simulink library "modbus_lib"  (R2016b)
settings: Solver=ode45  StartTime=0.0  StopTime=10.0  RelTol=1e-3  EnableMultiTasking=on
undefined symbols (not defined in the file): angle_threshold, dF_threshold, DiscIntNeverNeededParam, dV_threshold, IOC, relay_sets, TOC, Ts, V, VRMSLL
libraries: simulink x21, powerlib_extras x20, powerlib x20, modbus_lib x8, simulink_extras x5, lib_Timer_Counter x4, rtio_generic_modbus x3, simulink_need_slupdate x3, dspsigops x2, discreteBreakerBlock x1
(part 1 of 2)
settings Model: Creator=RE25624  LastModifiedBy=ch24070
settings DataIOCC: LimitDataPoints=on  SaveFormat=Array  SignalLoggingSaveFormat=ModelDataLogs
settings OptimizationCC: ExpressionDepthLimit=2147483647  LifeSpan=inf
settings DebuggingCC: UnderspecifiedInitializationDetection=Classic  MergeDetectMultiDrivingBlocksExec=none  SolverPrmCheckMsg=warning  FcnCallInpInsideContextMsg=warning  StateNameClashWarn=warning  SFUnexpectedBacktrackingDiag=warning  SFNoUnconditionalDefaultTransitionDiag=warning  SFExecutionAtInitializationDiag=none
settings HardwareCC: ProdBitPerPointer=32  ProdBitPerSizeT=32  ProdBitPerPtrDiffT=32  ProdLargestAtomicFloat=None  ProdIntDivRoundTo=Undefined  ProdEndianess=Unspecified  ProdWordSize=32  ProdHWDeviceType=32-bit Generic
settings ModelReferenceCC: PropagateSignalLabelsOutOfModel=off
settings GRTTargetCC: TargetLangStandard=C89/C90 (ANSI)  GeneratePreprocessorConditionals=Disable all  CombineOutputUpdateFcns=off  GRTInterface=on
settings ConfigComp: CovMetricSettings=dw  CovHtmlReporting=on  CovSaveCumulativeToWorkspaceVar=on  CovSaveSingleToWorkspaceVar=on  CovExternalEMLEnable=off

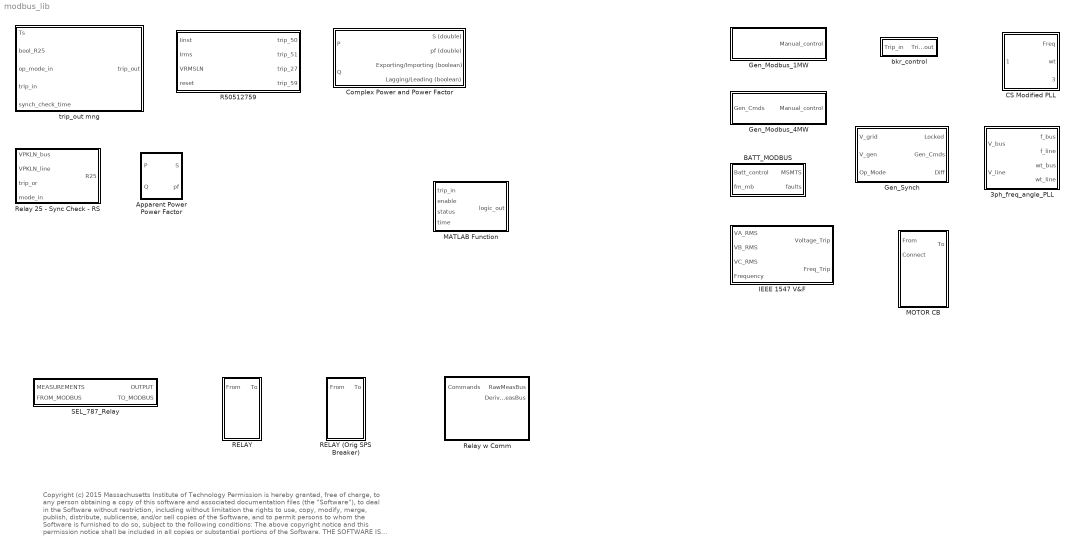
== system modbus_lib ==
  note: Copyright (c) 2015 Massachusetts Institute of Technology
      | Permission is hereby granted, free of charge, to any person obtaining a copy of this software and associated documentation files (the "Software"), to deal in the Software without restriction, including without limitation the rights to use, copy, modify, merge, publish, distribute, sublicense, and/or sell copies of the Software, and to permit persons to whom the Software is furnished to do so, subject to the following conditions:
      |
      | The above copyright notice and this permission notice shall be included in all copies or substantial portions of the Software.
      |
      | THE SOFTWARE IS PROVIDED "AS IS", WITHOUT WARRANTY OF ANY KIND, EXPRESS OR IMPLIED, INCLUDING BUT NOT LIMITED TO THE WARRANTIES OF MERCHANTABILITY, FITNESS FOR A PARTICULAR PURPOSE AND NONINFRINGEMENT. IN NO EVENT SHALL THE AUTHORS OR COPYRIGHT HOLDERS BE LIABLE FOR ANY CLAIM,
      | DAMAGES OR OTHER LIABILITY, WHETHER IN AN ACTION OF CONTRACT, TORT OR OTHERWISE, ARISING FROM, OUT OF OR IN CONNECTION WITH THE SOFTWARE OR THE USE OR OTHER DEALINGS IN THE SOFTWARE.
  3ph_freq_angle_PLL : Subsystem
  Apparent Power Power Factor : Subsystem
  BATT_MODBUS : Subsystem
  CS Modified PLL : Subsystem  DialogController=POWERSYS.PowerSysDialog  mask(Discrete 3-phase PLL){Fmin=50, Par_Init=[0 60], ParK=[ 180 3200 1 ], Ts=Ts, AGC=off}
      mask prompts: Fmin "Minimum frequency (Hz):"; Par_Init "Initial inputs:[ Phase(degrees)   Frequency(Hz) ]"; ParK "Regulator gains [ Kp  Ki  Kd ]"; Ts "Sample time:"; AGC "Enable Automatic Gain Control"
      mask help:
      | This Phase Locked Loop (PLL) system can be used  to synchronize on a set of variable frequency, three-phase sinusoidal signals. If the Automatic Gain Control is enabled, the input (phase error) of the PLL regulator is scaled according to the input signals magnitude.
      |
      | For optimal performance, the following settings are recommended:
      |   [ Kp Ki  Kd ] = [ 180  3200  1 ]
      |   "Enable Automatic Gain Control" checked
      |
      | Input 1: Vector containing the normalized three-phase signals [Va Vb Vc]
      | Output 1:  Measured frequency (Hz) = w/(2pi)
      | Output 2:  Ramp w.t varying between  0 and 2*pi,
      |      synchronized on zero crossings of the fundamental (positive-sequence) of phase A.
      | Output 3: Vector [sin(wt) cos(wt)]
      mask init:
      | Kp=ParK(1);
      | Ki=ParK(2);
      | if length(ParK)==2
      |     Kd=0;
      | else
      |     Kd=ParK(3);
      | end    
      | Phase_Init=Par_Init(1);
      | Finit=Par_Init(2);
      | power_initmask();
      settings: OpenFcn=power_openblockproxy();
      mask Display: disp('')
  Complex Power and Power Factor : Subsystem
  Gen_Modbus_1MW : Subsystem
  Gen_Modbus_4MW : Subsystem
  Gen_Synch : Subsystem
  IEEE 1547 V&F : Subsystem  mask{V=VRMSLL, OF1=2, OF2=0.16, OV1=13, OV2=0.16, UF1=0.16, UF2=2, UV1=0.16, UV2=11, UV3=21}
      mask prompts: V "VoltageLL_RMS"; OF1 "OF1 (>60.5 Hz)"; OF2 "OF2 (>62 Hz)"; OV1 "OV1 (110% <V< 120% Vnom"; OV2 "OV2 (120% Vnom)"; UF1 "UF1 (<57 Hz)"; UF2 "UF2 (<59.5 Hz)"; UV1 "UV1 (<45% Vnom)"; UV2 "UV2 (45%<V<60% Vnom)"; UV3 "UV3 (60%<V<88% Vnom)"
      mask help:
      | This block implements interconnection system response according to IEEE Std. 1547-2014a.
      |
      | Fields to be filled are clearing times in seconds.
      mask TypeOptions V: Vnom/Value
      mask TypeOptions OF1: OF1/Value
      mask TypeOptions OF2: OF2/Value
      mask TypeOptions OV1: OV1/Value
      mask TypeOptions OV2: OV2/Value
      mask TypeOptions UF1: UF1/Value
      mask TypeOptions UF2: UF2/Value
      mask TypeOptions UV1: UV1/Value
      mask TypeOptions UV2: UV2/Value
      mask TypeOptions UV3: UV3/Value
  MATLAB Function : MATLAB Function  TreatAsAtomicUnit=on
  MOTOR CB : Subsystem  mask(Breaker){Ts=Ts}
      mask prompts: Ts "Sampling Time [Sec]"
      mask help:
      | This block simulates the open/close behavior of a breaker. The logic (1-closed; 0-open) of operation is provided via external relay-blocks.
      | The breaker model also facilitates the system measurements for all logic functions to operate.
      | The connectivity convention adopted for this block is as follows: ABC indicates the “entry-point” or line, and the abc indicates the “exit-point” or bus.
  R50512759 : Subsystem  mask(Relays 50-51-27-59){VRMSLL=VRMSLL, IOC=IOC, TOC=TOC, Ts=Ts}
      mask prompts: VRMSLL "Nominal Voltage [VRMSLL]"; IOC "IOC Setting [A]"; TOC "TOC Setting [A]"; Ts "Sampling Time [Sec]"
      mask help:
      | This block simulates the behavior of the following relay functions:
      | 1) Instantaneous overcurrent (50)
      | 2) AC inverse time overcurrent (51)
      | 3) Undervoltage (27)
      | 4) Overvoltage (59)
      | It is not suitable for instantaneous earth current relaying.
      | The model neglects the influence CTs since only the logics of the relay are required or the current effort.
  RELAY : Subsystem  mask(Breaker){Ts=Ts}
      mask prompts: Ts "Sampling Time [Sec]"
      mask help:
      | This block simulates the open/close behavior of a breaker. The logic (1-closed; 0-open) of operation is provided via external relay-blocks.
      | The breaker model also facilitates the system measurements for all logic functions to operate.
      | The connectivity convention adopted for this block is as follows: ABC indicates the “entry-point” or line, and the abc indicates the “exit-point” or bus.
  RELAY (Orig SPS Breaker) : Subsystem  mask(Breaker){Ts=Ts}
      mask prompts: Ts "Sampling Time [Sec]"
      mask help:
      | This block simulates the open/close behavior of a breaker. The logic (1-closed; 0-open) of operation is provided via external relay-blocks.
      | The breaker model also facilitates the system measurements for all logic functions to operate.
      | The connectivity convention adopted for this block is as follows: ABC indicates the “entry-point” or line, and the abc indicates the “exit-point” or bus.
  Relay 25 - Sync Check - RS : Subsystem  mask{VRMSLL=VRMSLL, Ts=Ts, dV_threshold=dV_threshold, angle_threshold=angle_threshold, dF_threshold=dF_threshold}
      mask prompts: VRMSLL "Nominal Voltage [VRMSLL]"; Ts "Sampling Time [Sec]"; dV_threshold "Percent Voltage Threshold [%]"; angle_threshold "Angle Threshold [degress]"; dF_threshold "Frequency Threshold [Hz]"
  Relay w Comm : Subsystem
  SEL_787_Relay : Subsystem  mask(Relay Model){bkrCtrl_enable=0, bkrCtrl_status=1, settings=[relay_sets(1, :)], Ts=Ts}
      mask prompts: bkrCtrl_enable "Enable - manual breaker control"; bkrCtrl_status "Status - manual breaker control"; settings "Relay Settings [Vnom(VRMSLL) IOC(A) TOC(A) dV(%)  dA(degrees)  dF(Hz)]"; Ts "Sampling Time [Sec]"
      mask help:
      | * The simulated relay functions are the following: synchronizing or synchronism-check (25), phase instantaneous overcurrent (50P), AC inverse time overcurrent (51P), undervoltage relay (27), and overvoltage relay (59).
      | * Modbus communication
      | * Locked-out only enabled for functions (50), (51)
      | * Over/undervoltage settings are set to +-15% of nominal voltage
      | * Manual breaker status: [1-closed, 0-open]
      mask init:
      | VRMSLL = settings(1);
      | IOC = settings(2);
      | TOC = settings(3);
      | dV_threshold = settings(4)/100;
      | angle_threshold = settings(5);
      | dF_threshold = settings(6);
  bkr_control : Subsystem  mask(Breaker control){enable=0, status=1}
      mask prompts: status "Breaker status: [1-closed, 0-open]"
      mask help: Allows the user to select which trip signal will be received at the breaker.
  trip_out mng : MATLAB Function  TreatAsAtomicUnit=on

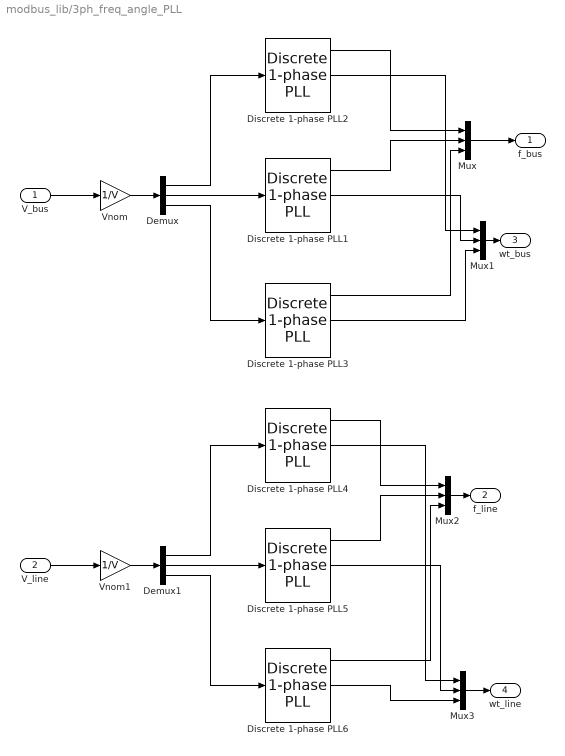
== system modbus_lib/3ph_freq_angle_PLL ==
  V_bus : Inport
  V_line : Inport  Port=2
  Demux : Demux  Outputs=3
  Demux1 : Demux  Outputs=3
  Discrete 1-phase PLL{1..6} (6 alike) : powerlib_extras/Discrete  Control Blocks/Discrete 1-phase PLL  Fmin=45  Par_Init=[0 60]  ParK=[ 180 3200 1]  Ts=50e-6  AGC=on
  Mux{,1..3} (4 alike) : Mux  Inputs=3
  Vnom : Gain  Gain=1/V
  Vnom1 : Gain  Gain=1/V
  f_bus : Outport
  f_line : Outport  Port=2
  wt_bus : Outport  Port=3
  wt_line : Outport  Port=4
  wires:
  V_bus/1 -> Vnom/1
  Mux3/1 -> wt_line/1
  Mux2/1 -> f_line/1
  Discrete 1-phase PLL6/2 -> Mux3/3
  Discrete 1-phase PLL5/2 -> Mux3/2
  Discrete 1-phase PLL4/2 -> Mux3/1
  Discrete 1-phase PLL5/1 -> Mux2/2
  Discrete 1-phase PLL6/1 -> Mux2/3
  Discrete 1-phase PLL4/1 -> Mux2/1
  Mux1/1 -> wt_bus/1
  Discrete 1-phase PLL3/2 -> Mux1/3
  Discrete 1-phase PLL1/2 -> Mux1/2
  Discrete 1-phase PLL2/2 -> Mux1/1
  Mux/1 -> f_bus/1
  Discrete 1-phase PLL3/1 -> Mux/3
  Discrete 1-phase PLL1/1 -> Mux/2
  Discrete 1-phase PLL2/1 -> Mux/1
  Demux/3 -> Discrete 1-phase PLL3/1
  Demux/2 -> Discrete 1-phase PLL1/1
  Demux/1 -> Discrete 1-phase PLL2/1
  Demux1/3 -> Discrete 1-phase PLL6/1
  Demux1/2 -> Discrete 1-phase PLL5/1
  Demux1/1 -> Discrete 1-phase PLL4/1
  Vnom1/1 -> Demux1/1
  Vnom/1 -> Demux/1
  V_line/1 -> Vnom1/1

== system modbus_lib/Apparent Power Power Factor ==
  note: Limit pf -1 -> 1
  note: Jason LaPenta
      | Sept 14, 2015
      |
      | Calculates 4 quadrant power factor and apparent power.
      | Both P and Q have valid negative values. At the PCC
      | both P and Q may be imported or exported.
  P : Inport
  Q : Inport  Port=2
  Constant : Constant  Value=pi/2
  Constant1 : Constant  Value=pi/2
  Constant2 : Constant  Value=2
  Divide : Product  Inputs=*/
  Divide1 : Product  Inputs=*/
  Divide2 : Product  Inputs=*/
  Sum : Sum  Inputs=|-+
  Sum1 : Sum  Inputs=|-+
  Switch : Switch  Criteria=u2 > Threshold  Threshold=1
  Trigonometric Function : Trigonometry  Operator=atan
  Trigonometric Function1 : Trigonometry  Operator=cos
  S : Outport
  pf : Outport  Port=2
  wires:
  Switch/1 -> pf/1
  Constant2/1 -> Sum1/1
  Sum1/1 -> Switch/1
  Divide1/1 -> Switch/3, Switch/2, Sum1/2
  Sum/1 -> Divide1/1
  Constant1/1 -> Sum/2
  Divide2/1 -> S/1
  Trigonometric Function1/1 -> Divide2/2
  Constant/1 -> Divide1/2
  Trigonometric Function/1 -> Sum/1, Trigonometric Function1/1  "theta"
  Divide/1 -> Trigonometric Function/1
  P/1 -> Divide2/1, Divide/2
  Q/1 -> Divide/1

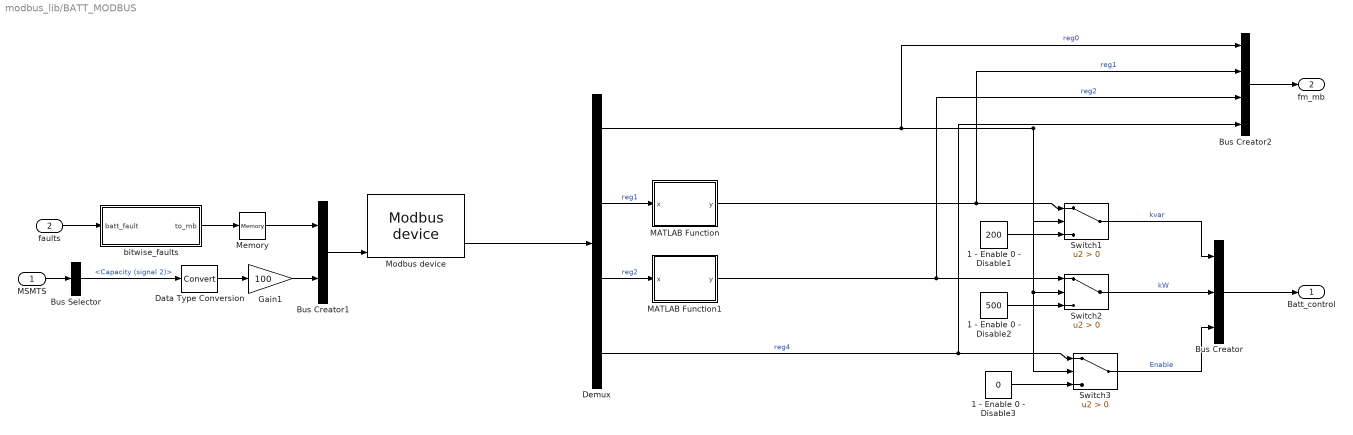
== system modbus_lib/BATT_MODBUS ==
  MSMTS : Inport
  faults : Inport  Port=2
  1 - Enable 0 - Disable1 : Constant  Value=200
  1 - Enable 0 - Disable2 : Constant  Value=500
  1 - Enable 0 - Disable3 : Constant  Value=0
  Bus Creator : BusCreator  Inputs=3
  Bus Creator1 : BusCreator  Inputs=2
  Bus Creator2 : BusCreator  Inputs=4
  Bus Selector : BusSelector  OutputSignals=Capacity (signal 2)
  Data Type Conversion : DataTypeConversion
  Demux : Demux
  Gain1 : Gain  Gain=100
  MATLAB Function : MATLAB Function  TreatAsAtomicUnit=on
  MATLAB Function1 : MATLAB Function  TreatAsAtomicUnit=on
  Memory : Memory
  Modbus device : rtio_generic_modbus/Modbus device  conf_name=batt_slave_cfg.opal  conf_name_mask=batt_slave_cfg.xls  sample_time=Ts
  Switch1 : Switch  Criteria=u2 > Threshold
  Switch2 : Switch  Criteria=u2 > Threshold
  Switch3 : Switch  Criteria=u2 > Threshold
  bitwise_faults : Subsystem
  Batt_control : Outport
  fm_mb : Outport  Port=2
  wires:
  MATLAB Function/1(y) -> Bus Creator2/2, Switch1/1  "reg1"
  MATLAB Function1/1(y) -> Bus Creator2/3, Switch2/1  "reg2"
  Memory/1 -> Bus Creator1/1
  faults/1 -> bitwise_faults/1(batt_fault)
  bitwise_faults/1(to_mb) -> Memory/1
  Bus Creator2/1 -> fm_mb/1
  Gain1/1 -> Bus Creator1/2
  Bus Creator1/1 -> Modbus device/4
  Data Type Conversion/1 -> Gain1/1
  Bus Selector/1 -> Data Type Conversion/1  "<Capacity (signal 2)>"
  MSMTS/1 -> Bus Selector/1
  Bus Creator/1 -> Batt_control/1
  Switch3/1 -> Bus Creator/3  "Enable"
  Switch2/1 -> Bus Creator/2  "kW"
  Switch1/1 -> Bus Creator/1  "kvar"
  Demux/1 -> Bus Creator2/1, Switch3/2, Switch2/2, Switch1/2  "reg0"
  Demux/4 -> Bus Creator2/4, Switch3/1  "reg4"
  Demux/3 -> MATLAB Function1/1(x)  "reg2"
  Demux/2 -> MATLAB Function/1(x)  "reg1"
  1 - Enable 0 - Disable3/1 -> Switch3/3
  1 - Enable 0 - Disable2/1 -> Switch2/3
  1 - Enable 0 - Disable1/1 -> Switch1/3
  Modbus device/2 -> Demux/1

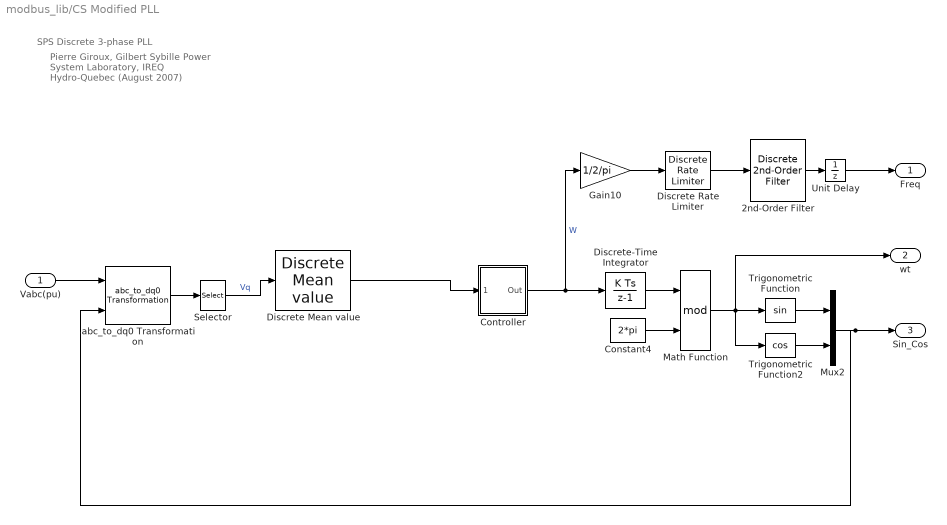
== system modbus_lib/CS Modified PLL ==
  note: Pierre Giroux, Gilbert Sybille
      | Power System Laboratory, IREQ
      | Hydro-Quebec
      | (August 2007)
  note: SPS Discrete 3-phase PLL
  Vabc(pu) : Inport  PortDimensions=3
  2nd-Order Filter : powerlib_extras/Discrete  Control Blocks/Discrete  2nd-Order Filter  FilterType=Lowpass  Fo=25  Zeta=0.707  Ts=Ts  Initialize=on  Vac_Init=[0 0 Finit]  Vdc_Init=Finit  PlotResponse=off  param1=[1 500 0.1]
  Constant4 : Constant  Value=2*pi
  Controller : Subsystem  mask(Discrete PID Controller){Kp=Kp, Ki=Ki, Kd=Kd, Par_Limits=[10000 0], Init=2*pi*Finit, Ts=Ts}
      mask prompts: Kp "Proportional gain (Kp):"; Ki "Integral gain (Ki):"; Kd "Derivative gain (Kd):"; Par_Limits "Output limits: [ Upper   Lower ]"; Init "Output initial value:"; Ts "Sample time:"
      mask help: This block implements a discrete PID controller.
      mask init:
      | UpperLimit=Par_Limits(1);
      | LowerLimit=Par_Limits(2);
      | power_initmask();
      settings: OpenFcn=power_openblockproxy();
      mask Display: disp('PID');
  Discrete Rate Limiter : powerlib_extras/Discrete  Control Blocks/Discrete Rate Limiter  R=12  F=-12  Vinit=Finit  Ts=Ts
  Discrete Mean value : powerlib_extras/Discrete Measurements/Discrete  Mean value  Freq=60  Vinit=0  Ts=Ts
  Discrete-Time Integrator : DiscreteIntegrator  InitialCondition=Phase_Init*pi/180  SampleTime=Ts  ICPrevOutput=DiscIntNeverNeededParam  ICPrevScaledInput=DiscIntNeverNeededParam
  Gain10 : Gain  Gain=1/2/pi  SaturateOnIntegerOverflow=on  OutDataTypeStr=Inherit: Same as input  ParamDataTypeStr=Inherit: Same as input
  Math Function : Math  Operator=mod  SaturateOnIntegerOverflow=on
  Mux2 : Mux  Inputs=2
  Selector : Selector  InputPortWidth=3  IndexOptions=Index vector (dialog)  Indices=2  OutputSizes=1
  Trigonometric Function : Trigonometry
  Trigonometric Function2 : Trigonometry  Operator=cos
  Unit Delay : UnitDelay  InitialCondition=Finit  SampleTime=Ts
  abc_to_dq0 Transformation : powerlib_extras/Measurements/abc_to_dq0 Transformation
  Freq : Outport
  wt : Outport  Port=2
  Sin_Cos : Outport  Port=3
  wires:
  Selector/1 -> Discrete Mean value/1  "Vq"
  2nd-Order Filter/1 -> Unit Delay/1
  Unit Delay/1 -> Freq/1
  Discrete Rate Limiter/1 -> 2nd-Order Filter/1
  Gain10/1 -> Discrete Rate Limiter/1
  Mux2/1 -> Sin_Cos/1, abc_to_dq0 Transformation/2
  Trigonometric Function2/1 -> Mux2/2
  Trigonometric Function/1 -> Mux2/1
  Math Function/1 -> Trigonometric Function/1, wt/1, Trigonometric Function2/1
  Discrete-Time Integrator/1 -> Math Function/1
  Constant4/1 -> Math Function/2
  abc_to_dq0 Transformation/1 -> Selector/1
  Vabc(pu)/1 -> abc_to_dq0 Transformation/1
  Controller/1(Out) -> Discrete-Time Integrator/1, Gain10/1  "W"
  Discrete Mean value/1 -> Controller/1(Error)

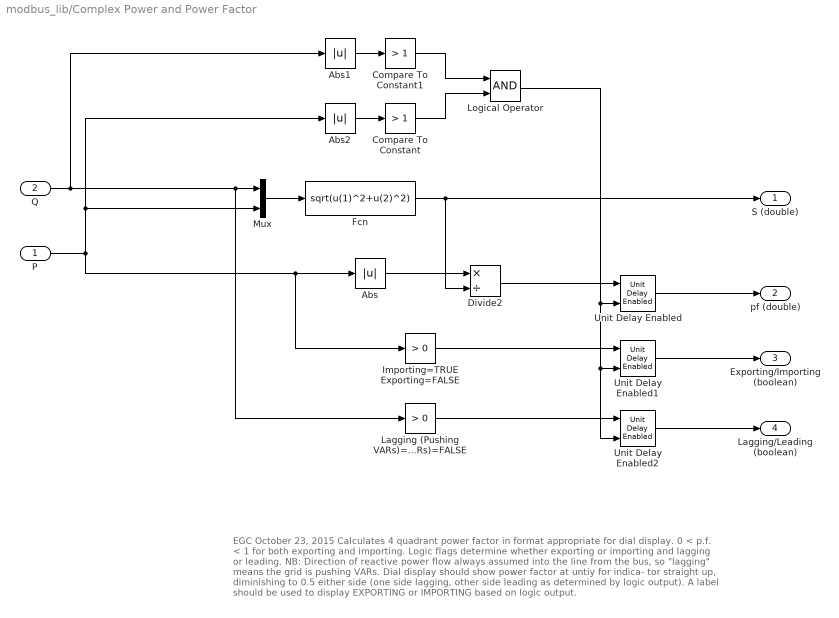
== system modbus_lib/Complex Power and Power Factor ==
  note: EGC
      | October 23, 2015
      |
      | Calculates 4 quadrant power factor in format appropriate
      | for dial display.  0 < p.f. < 1 for both exporting and
      | importing.  Logic flags determine whether exporting or
      | importing and lagging or leading.  NB:  Direction of
      | reactive power flow always assumed into the line from the
      | bus, so "lagging" means the grid is pushing VARs.
      |
      | Dial display should show power factor at untiy for indica-
      | tor straight up, diminishing to 0.5 either side (one side
      | lagging, other side leading as determined by logic output).
      | A label should be used to display EXPORTING or IMPORTING
      | based on logic output.
  P : Inport
  Q : Inport  Port=2
  Abs : Abs
  Abs1 : Abs
  Abs2 : Abs
  Compare To Constant : simulink/Logic and Bit Operations/Compare To Constant  relop=>  const=1  OutDataTypeStr=uint8
  Compare To Constant1 : simulink/Logic and Bit Operations/Compare To Constant  relop=>  const=1  OutDataTypeStr=uint8
  Divide2 : Product  Inputs=*/
  Fcn : Fcn  Expr=sqrt(u(1)^2+u(2)^2)
  Importing=TRUE Exporting=FALSE : simulink/Logic and Bit Operations/Compare To Constant  relop=>  const=0  OutDataTypeStr=boolean
  Lagging (Pushing VARs)=TRUE Leading (Pulling VARs)=FALSE : simulink/Logic and Bit Operations/Compare To Constant  relop=>  const=0  OutDataTypeStr=boolean
  Logical Operator : Logic  AllPortsSameDT=off  OutDataTypeStr=boolean
  Mux : Mux  Inputs=2
  Unit Delay Enabled : simulink_need_slupdate/Unit Delay Enabled  vinit=1  tsamp=-1
  Unit Delay Enabled1 : simulink_need_slupdate/Unit Delay Enabled  vinit=1  tsamp=-1
  Unit Delay Enabled2 : simulink_need_slupdate/Unit Delay Enabled  vinit=1  tsamp=-1
  S (double) : Outport
  pf (double) : Outport  Port=2
  Exporting/Importing (boolean) : Outport  Port=3
  Lagging/Leading (boolean) : Outport  Port=4
  wires:
  Fcn/1 -> Divide2/2, S (double)/1
  P/1 -> Abs/1, Importing=TRUE Exporting=FALSE/1, Mux/2, Abs2/1
  Q/1 -> Mux/1, Lagging (Pushing VARs)=TRUE Leading (Pulling VARs)=FALSE/1, Abs1/1
  Mux/1 -> Fcn/1
  Abs/1 -> Divide2/1
  Divide2/1 -> Unit Delay Enabled/1
  Unit Delay Enabled/1 -> pf (double)/1
  Importing=TRUE Exporting=FALSE/1 -> Unit Delay Enabled1/1
  Unit Delay Enabled1/1 -> Exporting/Importing (boolean)/1
  Lagging (Pushing VARs)=TRUE Leading (Pulling VARs)=FALSE/1 -> Unit Delay Enabled2/1
  Unit Delay Enabled2/1 -> Lagging/Leading (boolean)/1
  Abs2/1 -> Compare To Constant/1
  Abs1/1 -> Compare To Constant1/1
  Compare To Constant1/1 -> Logical Operator/1
  Compare To Constant/1 -> Logical Operator/2
  Logical Operator/1 -> Unit Delay Enabled/2, Unit Delay Enabled1/2, Unit Delay Enabled2/2

== system modbus_lib/Gen_Modbus_1MW ==
  note: This function is an attempt to substitute the switches
  Bus Creator : BusCreator  Inputs=6
  Demux : Demux  Outputs=7
  Gain : Gain  Gain=1/100
  MATLAB Function : MATLAB Function  TreatAsAtomicUnit=on
  Modbus device : rtio_generic_modbus/Modbus device  conf_name=none  conf_name_mask=gen_slave_cfg2.xls  sample_time=Ts
  Manual_control : Outport
  wires:
  Gain/1 -> Demux/1
  Modbus device/2 -> Gain/1
  Demux/1 -> MATLAB Function/1(Select_mb)
  Demux/2 -> MATLAB Function/2(P_mb)
  Demux/3 -> MATLAB Function/3(Q_mb)
  Demux/4 -> MATLAB Function/4(V_mb)
  Demux/5 -> MATLAB Function/5(F_mb)
  Demux/6 -> MATLAB Function/6(Mode_mb)
  Demux/7 -> MATLAB Function/7(Enable_mb)
  Bus Creator/1 -> Manual_control/1
  MATLAB Function/1(P) -> Bus Creator/1  "P"
  MATLAB Function/2(Q) -> Bus Creator/2  "Q"
  MATLAB Function/3(V) -> Bus Creator/3  "V"
  MATLAB Function/4(F) -> Bus Creator/4  "F"
  MATLAB Function/5(Mode) -> Bus Creator/5  "Mode"
  MATLAB Function/6(Enable) -> Bus Creator/6  "Enable"

== system modbus_lib/Gen_Modbus_4MW ==
  note: This function is an attempt to substitute the switches
  Gen_Cmds : Inport
  Bus Creator : BusCreator  Inputs=6
  Demux : Demux  Outputs=7
  Gain : Gain  Gain=1/100
  MATLAB Function : MATLAB Function  TreatAsAtomicUnit=on
  Modbus device : rtio_generic_modbus/Modbus device  conf_name=gen_slave_cfg.opal  conf_name_mask=gen_slave_cfg.xls  sample_time=Ts
  Manual_control : Outport
  wires:
  Gain/1 -> Demux/1
  Demux/1 -> MATLAB Function/1(Select_mb)
  Demux/2 -> MATLAB Function/2(P_mb)
  Demux/3 -> MATLAB Function/3(Q_mb)
  Demux/4 -> MATLAB Function/4(V_mb)
  Demux/5 -> MATLAB Function/5(F_mb)
  Demux/6 -> MATLAB Function/6(Mode_mb)
  Demux/7 -> MATLAB Function/7(Enable_mb)
  Bus Creator/1 -> Manual_control/1
  MATLAB Function/1(P) -> Bus Creator/1  "P"
  MATLAB Function/2(Q) -> Bus Creator/2  "Q"
  MATLAB Function/3(V) -> Bus Creator/3  "V"
  MATLAB Function/4(F) -> Bus Creator/4  "F"
  MATLAB Function/5(Mode) -> Bus Creator/5  "Mode"
  MATLAB Function/6(Enable) -> Bus Creator/6  "Enable"
  Modbus device/2 -> Gain/1
  Gen_Cmds/1 -> MATLAB Function/8(gen_cmds)

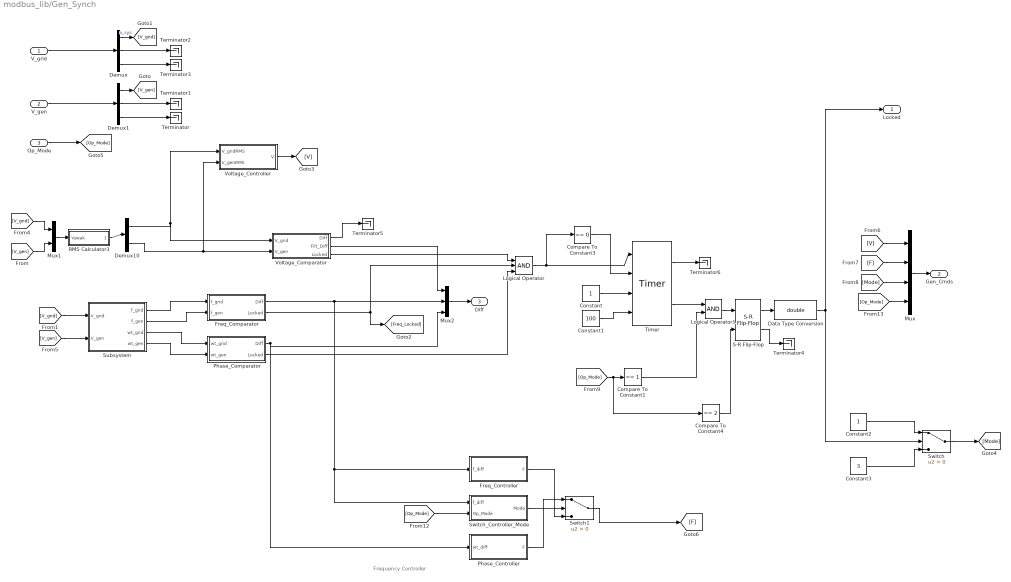
== system modbus_lib/Gen_Synch ==
  note: Frequency Controller
  V_grid : Inport
  V_gen : Inport  Port=2
  Op_Mode : Inport  Port=3
  Compare To Constant1 : simulink/Logic and Bit Operations/Compare To Constant  relop===  const=1  OutDataTypeStr=boolean
  Compare To Constant3 : simulink/Logic and Bit Operations/Compare To Constant  relop===  const=0  OutDataTypeStr=uint8
  Compare To Constant4 : simulink/Logic and Bit Operations/Compare To Constant  relop===  const=2  OutDataTypeStr=boolean
  Constant : Constant
  Constant1 : Constant  Value=100
  Constant2 : Constant
  Constant3 : Constant  Value=3
  Data Type Conversion : DataTypeConversion  OutDataTypeStr=double
  Demux : Demux  Outputs=3
  Demux1 : Demux  Outputs=3
  Demux10 : Demux  Outputs=2
  Freq_Comparator : Subsystem
  Freq_Controller : Subsystem
  Logical Operator : Logic  Inputs=3  AllPortsSameDT=off  OutDataTypeStr=boolean
  Logical Operator1 : Logic  AllPortsSameDT=off  OutDataTypeStr=boolean
  Mux : Mux
  Mux1 : Mux  Inputs=2
  Mux2 : Mux  Inputs=3
  Phase_Comparator : Subsystem
  Phase_Controller : Subsystem
  RMS Calculator3 : Subsystem
  S-R Flip-Flop : simulink_extras/Flip Flops/S-R Flip-Flop  initial_condition=0
  Subsystem : Subsystem
  Switch : Switch  Criteria=u2 > Threshold
  Switch1 : Switch  Criteria=u2 > Threshold
  Switch_Controller_Mode : Subsystem
  Terminator{,1..6} (7 alike) : Terminator
  Timer : lib_Timer_Counter/Timer
  Voltage_Comparator : Subsystem
  Voltage_Controller : Subsystem
  Locked : Outport
  Gen_Cmds : Outport  Port=2  PortDimensions=4
  Diff : Outport  Port=3
  wires:
  Phase_Comparator/1(Diff) -> Mux2/3, Phase_Controller/1(wt_diff)
  Freq_Comparator/1(Diff) -> Mux2/2, Freq_Controller/1(f_diff), Switch_Controller_Mode/1(f_diff)
  Voltage_Comparator/2(Filt_Diff) -> Mux2/1
  [V_gen] -> Subsystem/2(V_gen)
  [V_grid] -> Subsystem/1(V_grid)
  Demux/1 -> [V_grid]  "a_sys"
  Demux1/1 -> [V_gen]
  Data Type Conversion/1 -> Switch/2, Locked/1
  S-R Flip-Flop/1 -> Data Type Conversion/1
  Logical Operator/1 -> Compare To Constant3/1, Timer/1
  Compare To Constant3/1 -> Timer/2
  Constant1/1 -> Timer/4
  Constant/1 -> Timer/3
  Phase_Comparator/2(Locked) -> Logical Operator/3
  Freq_Comparator/2(Locked) -> Logical Operator/2, [Freq_Locked]
  Voltage_Comparator/3(Locked) -> Logical Operator/1
  Subsystem/4(wt_gen) -> Phase_Comparator/2(wt_gen)
  Subsystem/3(wt_grid) -> Phase_Comparator/1(wt_grid)
  Subsystem/2(f_gen) -> Freq_Comparator/2(f_gen)
  Subsystem/1(f_grid) -> Freq_Comparator/1(f_grid)
  V_gen/1 -> Demux1/1
  V_grid/1 -> Demux/1
  Constant2/1 -> Switch/1
  Constant3/1 -> Switch/3
  Switch/1 -> [Mode]
  Mux/1 -> Gen_Cmds/1
  [V] -> Mux/1
  [Mode] -> Mux/3
  [F] -> Mux/2
  Timer/2 -> Logical Operator1/1
  Compare To Constant1/1 -> Logical Operator1/2
  Mux2/1 -> Diff/1
  Switch1/1 -> [F]
  Switch_Controller_Mode/1(Mode) -> Switch1/2
  Op_Mode/1 -> [Op_Mode]
  [Op_Mode] -> Compare To Constant1/1, Compare To Constant4/1
  Logical Operator1/1 -> S-R Flip-Flop/1
  Compare To Constant4/1 -> S-R Flip-Flop/2
  [Op_Mode] -> Mux/4
  Voltage_Controller/1(V) -> [V]
  Freq_Controller/1(F) -> Switch1/3
  Phase_Controller/1(F) -> Switch1/1
  [Op_Mode] -> Switch_Controller_Mode/2(Op_Mode)
  Demux1/2 -> Terminator1/1
  Demux1/3 -> Terminator/1
  Demux/2 -> Terminator2/1
  Demux/3 -> Terminator3/1
  S-R Flip-Flop/2 -> Terminator4/1
  Voltage_Comparator/1(Diff) -> Terminator5/1
  Demux10/2 -> Voltage_Comparator/2(V_gen), Voltage_Controller/2(V_genRMS)
  Mux1/1 -> RMS Calculator3/1(Vpeak)
  RMS Calculator3/1(VRMSLL) -> Demux10/1
  [V_grid] -> Mux1/1
  [V_gen] -> Mux1/2
  Demux10/1 -> Voltage_Controller/1(V_gridRMS), Voltage_Comparator/1(V_grid)
  Timer/1 -> Terminator6/1

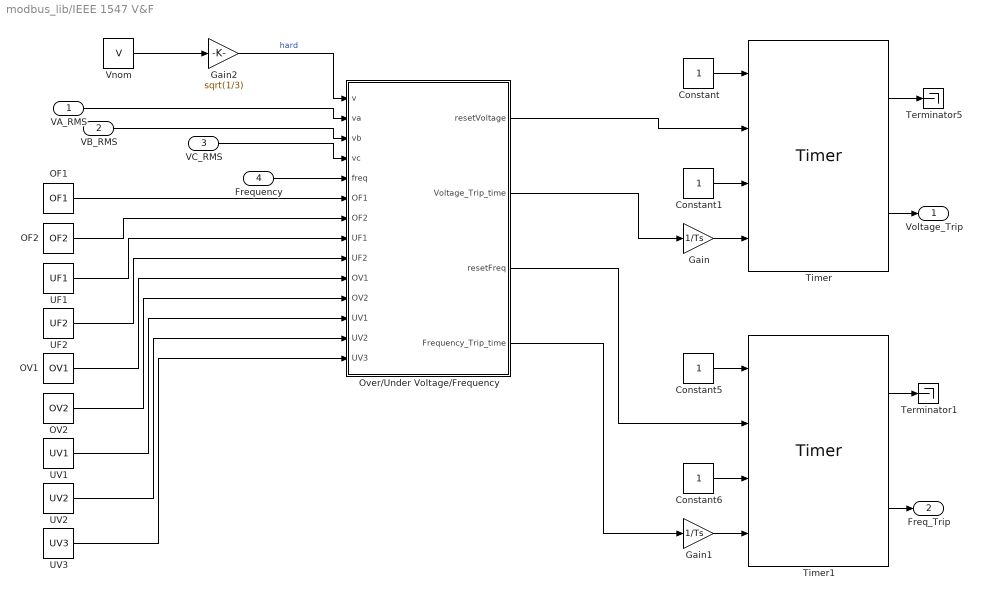
== system modbus_lib/IEEE 1547 V&F ==
  VA_RMS : Inport
  VB_RMS : Inport  Port=2
  VC_RMS : Inport  Port=3
  Frequency : Inport  Port=4
  Constant{,1,5..6} (4 alike) : Constant
  Gain : Gain  Gain=1/Ts
  Gain1 : Gain  Gain=1/Ts
  Gain2 : Gain  Gain=sqrt(1/3)
  OF1 : Constant  Value=OF1
  OF2 : Constant  Value=OF2
  OV1 : Constant  Value=OV1
  OV2 : Constant  Value=OV2
  Over/Under Voltage/Frequency : MATLAB Function  TreatAsAtomicUnit=on
  Terminator1 : Terminator
  Terminator5 : Terminator
  Timer : lib_Timer_Counter/Timer
  Timer1 : lib_Timer_Counter/Timer
  UF1 : Constant  Value=UF1
  UF2 : Constant  Value=UF2
  UV1 : Constant  Value=UV1
  UV2 : Constant  Value=UV2
  UV3 : Constant  Value=UV3
  Vnom : Constant  Value=V
  Voltage_Trip : Outport
  Freq_Trip : Outport  Port=2
  wires:
  UV3/1 -> Over/Under Voltage/Frequency/14(UV3)
  UV2/1 -> Over/Under Voltage/Frequency/13(UV2)
  UV1/1 -> Over/Under Voltage/Frequency/12(UV1)
  OV2/1 -> Over/Under Voltage/Frequency/11(OV2)
  OV1/1 -> Over/Under Voltage/Frequency/10(OV1)
  UF2/1 -> Over/Under Voltage/Frequency/9(UF2)
  UF1/1 -> Over/Under Voltage/Frequency/8(UF1)
  OF2/1 -> Over/Under Voltage/Frequency/7(OF2)
  OF1/1 -> Over/Under Voltage/Frequency/6(OF1)
  Gain/1 -> Timer/4
  Gain1/1 -> Timer1/4
  Frequency/1 -> Over/Under Voltage/Frequency/5(freq)
  VC_RMS/1 -> Over/Under Voltage/Frequency/4(vc)
  VB_RMS/1 -> Over/Under Voltage/Frequency/3(vb)
  Vnom/1 -> Gain2/1
  VA_RMS/1 -> Over/Under Voltage/Frequency/2(va)
  Timer1/2 -> Freq_Trip/1
  Constant6/1 -> Timer1/3
  Constant5/1 -> Timer1/1
  Constant1/1 -> Timer/3
  Constant/1 -> Timer/1
  Timer1/1 -> Terminator1/1
  Timer/1 -> Terminator5/1
  Timer/2 -> Voltage_Trip/1
  Over/Under Voltage/Frequency/1(resetVoltage) -> Timer/2
  Over/Under Voltage/Frequency/2(Voltage_Trip_time) -> Gain/1
  Over/Under Voltage/Frequency/4(Frequency_Trip_time) -> Gain1/1
  Over/Under Voltage/Frequency/3(resetFreq) -> Timer1/2
  Gain2/1 -> Over/Under Voltage/Frequency/1(v)  "hard"

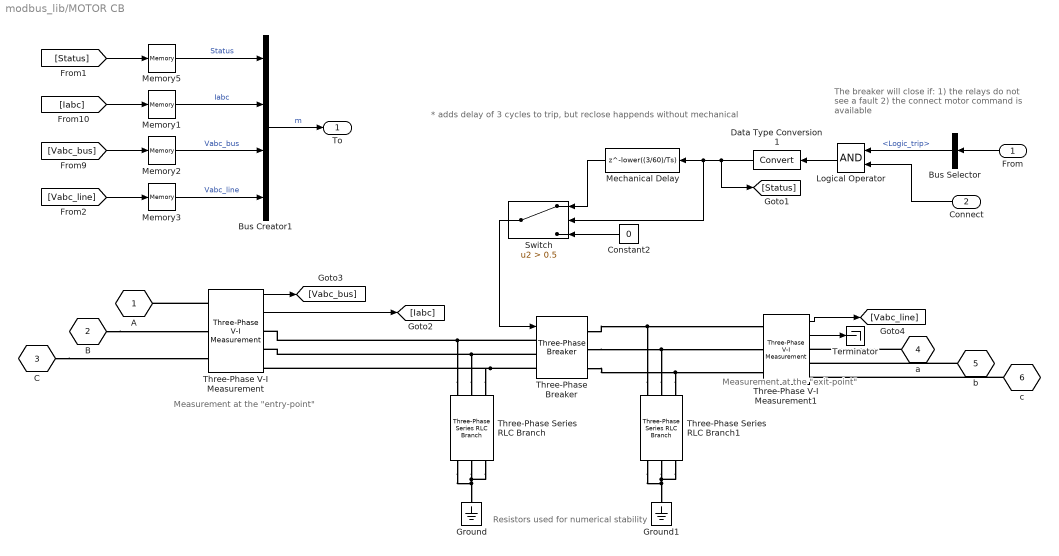
== system modbus_lib/MOTOR CB ==
  note: * adds delay of 3 cycles to trip, but reclose happends without mechanical
  note: Measurement at the "exit-point"
  note: Measurement at the "entry-point"
  note: Resistors used for numerical stability
  note: The breaker will close if:
      | 1) the relays do not see a fault
      | 2) the connect motor command is available
  From : Inport
  Connect : Inport  Port=2
  Bus Creator1 : BusCreator  Inputs=4
  Bus Selector : BusSelector  OutputSignals=Logic_trip
  Constant2 : Constant  Value=0
  Data Type Conversion1 : DataTypeConversion
  Ground : powerlib/Elements/Ground  LConnTagsString=a
  Ground1 : powerlib/Elements/Ground  LConnTagsString=a
  Logical Operator : Logic  AllPortsSameDT=off  OutDataTypeStr=boolean
  Mechanical Delay : Delay  DelayLength=lower((3/60)/Ts)  InitialCondition=1
  Memory{1..3,5} (4 alike) : Memory
  Switch : Switch  Criteria=u2 > Threshold  Threshold=0.5
  Terminator : Terminator
  Three-Phase Series RLC Branch : powerlib/Elements/Three-Phase Series RLC Branch  LConnTagsString=A|B|C  RConnTagsString=A|B|C  BranchType=R  Resistance=15E6  Inductance=1e-3  Capacitance=1e-6  Measurements=None
  Three-Phase Series RLC Branch1 : powerlib/Elements/Three-Phase Series RLC Branch  LConnTagsString=A|B|C  RConnTagsString=A|B|C  BranchType=R  Resistance=15E6  Inductance=1e-3  Capacitance=1e-6  Measurements=None
  Three-Phase V-I Measurement : powerlib/Measurements/Three-Phase V-I Measurement  VoltageMeasurement=phase-to-ground  SetLabelV=off  LabelV=Vabc  Vpu=off  VpuLL=off  CurrentMeasurement=yes  SetLabelI=off  LabelI=Iabc  Ipu=off  Pbase=100e6  Vbase=500e3  OutputType=Complex  PhasorSimulation=off  PSBequivalent=0
  Three-Phase V-I Measurement1 : powerlib/Measurements/Three-Phase V-I Measurement  VoltageMeasurement=phase-to-ground  SetLabelV=off  LabelV=Vabc  Vpu=off  VpuLL=off  CurrentMeasurement=yes  SetLabelI=off  LabelI=Iabc  Ipu=off  Pbase=100e6  Vbase=500e3  OutputType=Complex  PhasorSimulation=off  PSBequivalent=0
  Three-Phase Breaker : powerlib/Elements/Three-Phase Breaker  InitialState=open  SwitchA=on  SwitchB=on  SwitchC=on  SwitchTimes="[1/60  5/60]"  External=on  BreakerResistance=1e-4  SnubberResistance=1E15  SnubberCapacitance=inf  Measurements=None
  A : PMIOPort  Tag=PMCPort  Port=1  Side=Left
  B : PMIOPort  Tag=PMCPort  Port=2  Side=Left
  C : PMIOPort  Tag=PMCPort  Port=3  Side=Left
  a : PMIOPort  Tag=PMCPort  Port=4  Side=Right
  b : PMIOPort  Tag=PMCPort  Port=5  Side=Right
  c : PMIOPort  Tag=PMCPort  Port=6  Side=Right
  To : Outport
  wires:
  Constant2/1 -> Switch/3
  Mechanical Delay/1 -> Switch/1
  Switch/1 -> Three-Phase Breaker/1
  Memory3/1 -> Bus Creator1/4  "Vabc_line"
  Memory2/1 -> Bus Creator1/3  "Vabc_bus"
  Memory1/1 -> Bus Creator1/2  "Iabc"
  Memory5/1 -> Bus Creator1/1  "Status"
  Three-Phase V-I Measurement1/2 -> Terminator/1
  [Vabc_line] -> Memory3/1
  Three-Phase V-I Measurement1/1 -> [Vabc_line]
  From/1 -> Bus Selector/1
  [Vabc_bus] -> Memory2/1
  [Iabc] -> Memory1/1
  [Status] -> Memory5/1
  Data Type Conversion1/1 -> Switch/2, Mechanical Delay/1, [Status]
  Three-Phase V-I Measurement/2 -> [Iabc]
  Three-Phase V-I Measurement/1 -> [Vabc_bus]
  Bus Creator1/1 -> To/1  "m"
  Logical Operator/1 -> Data Type Conversion1/1
  Bus Selector/1 -> Logical Operator/1  "<Logic_trip>"
  Connect/1 -> Logical Operator/2
  connections:
  Three-Phase Series RLC Branch1/RConn1 -- Ground1/LConn1 -- Three-Phase Series RLC Branch1/RConn3 -- Three-Phase Series RLC Branch1/RConn2
  Three-Phase Series RLC Branch/RConn1 -- Ground/LConn1 -- Three-Phase Series RLC Branch/RConn3 -- Three-Phase Series RLC Branch/RConn2
  Three-Phase Series RLC Branch/LConn1 -- Three-Phase V-I Measurement/RConn1 -- Three-Phase Breaker/LConn1
  Three-Phase Series RLC Branch/LConn2 -- Three-Phase V-I Measurement/RConn2 -- Three-Phase Breaker/LConn2
  Three-Phase Series RLC Branch/LConn3 -- Three-Phase V-I Measurement/RConn3 -- Three-Phase Breaker/LConn3
  Three-Phase Series RLC Branch1/LConn1 -- Three-Phase V-I Measurement1/LConn1 -- Three-Phase Breaker/RConn1
  Three-Phase Series RLC Branch1/LConn2 -- Three-Phase V-I Measurement1/LConn2 -- Three-Phase Breaker/RConn2
  Three-Phase Series RLC Branch1/LConn3 -- Three-Phase V-I Measurement1/LConn3 -- Three-Phase Breaker/RConn3
  Three-Phase V-I Measurement/LConn1 -- A/RConn1
  B/RConn1 -- Three-Phase V-I Measurement/LConn2
  C/RConn1 -- Three-Phase V-I Measurement/LConn3
  a/RConn1 -- Three-Phase V-I Measurement1/RConn1
  b/RConn1 -- Three-Phase V-I Measurement1/RConn2
  c/RConn1 -- Three-Phase V-I Measurement1/RConn3

== system modbus_lib/R50512759 ==
  Iinst : Inport
  Irms : Inport  Port=2
  VRMSLN : Inport  Port=3
  reset : Inport  Port=4
  Data Type Conversion3 : DataTypeConversion
  Relays : MATLAB Function  TreatAsAtomicUnit=on
  a1 : Constant  Value=VRMSLL
  a2 : Constant  Value=TOC
  a4 : Constant  Value=Ts
  a5 : Constant  Value=IOC
  trip_50 : Outport
  trip_51 : Outport  Port=2
  trip_27 : Outport  Port=3
  trip_59 : Outport  Port=4
  wires:
  reset/1 -> Data Type Conversion3/1
  a5/1 -> Relays/6(IOC)  "IOC"
  Iinst/1 -> Relays/3(Iinst)
  a2/1 -> Relays/7(TOC)  "TOC"
  Irms/1 -> Relays/4(Irms)
  VRMSLN/1 -> Relays/5(Vrms)
  a1/1 -> Relays/8(VRMSLL)  "VRMSLL"
  a4/1 -> Relays/1(Ts)
  Relays/3(trip27) -> trip_27/1  "t27"
  Relays/4(trip59) -> trip_59/1  "t59"
  Relays/1(trip50) -> trip_50/1  "t50"
  Relays/2(trip51) -> trip_51/1  "t51"
  Data Type Conversion3/1 -> Relays/2(Reset)

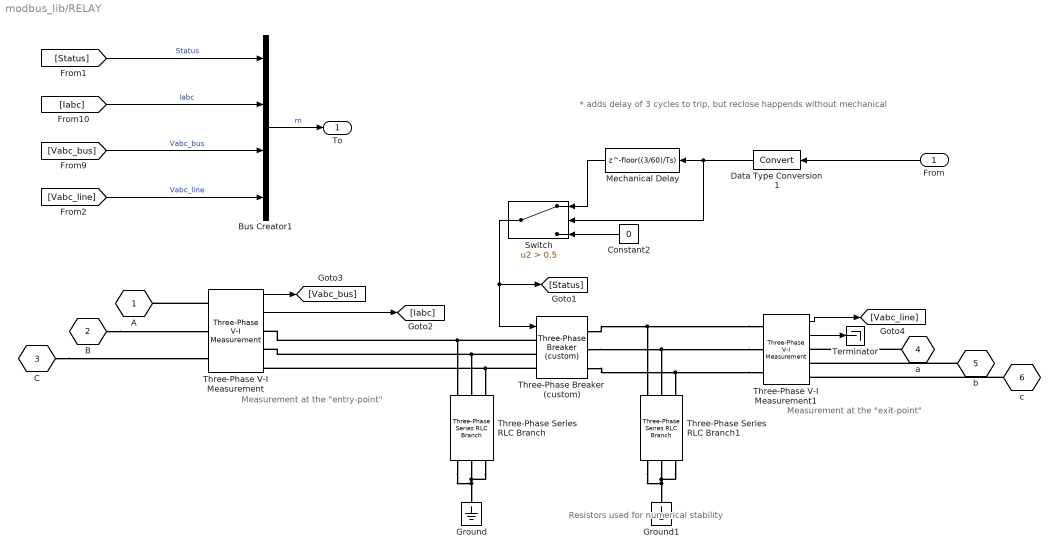
== system modbus_lib/RELAY ==
  note: Resistors used for numerical stability
  note: Measurement at the "entry-point"
  note: Measurement at the "exit-point"
  note: * adds delay of 3 cycles to trip, but reclose happends without mechanical
  From : Inport
  Bus Creator1 : BusCreator  Inputs=4
  Constant2 : Constant  Value=0
  Data Type Conversion1 : DataTypeConversion
  Ground : powerlib/Elements/Ground  LConnTagsString=a
  Ground1 : powerlib/Elements/Ground  LConnTagsString=a
  Mechanical Delay : Delay  DelayLength=floor((3/60)/Ts)  InitialCondition=1
  Switch : Switch  Criteria=u2 > Threshold  Threshold=0.5
  Terminator : Terminator
  Three-Phase Series RLC Branch : powerlib/Elements/Three-Phase Series RLC Branch  LConnTagsString=A|B|C  RConnTagsString=A|B|C  BranchType=R  Resistance=15E6  Inductance=1e-3  Capacitance=1e-6  Measurements=None
  Three-Phase Series RLC Branch1 : powerlib/Elements/Three-Phase Series RLC Branch  LConnTagsString=A|B|C  RConnTagsString=A|B|C  BranchType=R  Resistance=15E6  Inductance=1e-3  Capacitance=1e-6  Measurements=None
  Three-Phase V-I Measurement : powerlib/Measurements/Three-Phase V-I Measurement  VoltageMeasurement=phase-to-ground  SetLabelV=off  LabelV=Vabc  Vpu=off  VpuLL=off  CurrentMeasurement=yes  SetLabelI=off  LabelI=Iabc  Ipu=off  Pbase=100e6  Vbase=500e3  OutputType=Complex  PhasorSimulation=off  PSBequivalent=0
  Three-Phase V-I Measurement1 : powerlib/Measurements/Three-Phase V-I Measurement  VoltageMeasurement=phase-to-ground  SetLabelV=off  LabelV=Vabc  Vpu=off  VpuLL=off  CurrentMeasurement=yes  SetLabelI=off  LabelI=Iabc  Ipu=off  Pbase=100e6  Vbase=500e3  OutputType=Complex  PhasorSimulation=off  PSBequivalent=0
  Three-Phase Breaker (custom) : discreteBreakerBlock/Three-Phase Breaker (custom)  InitialState=closed  SwitchA=on  SwitchB=on  SwitchC=on  SwitchTimes=2/60  External=on  BreakerResistance=1e-4  SnubberResistance=1e15  SnubberCapacitance=inf  Measurements=None
  A : PMIOPort  Tag=PMCPort  Port=1  Side=Left
  B : PMIOPort  Tag=PMCPort  Port=2  Side=Left
  C : PMIOPort  Tag=PMCPort  Port=3  Side=Left
  a : PMIOPort  Tag=PMCPort  Port=4  Side=Right
  b : PMIOPort  Tag=PMCPort  Port=5  Side=Right
  c : PMIOPort  Tag=PMCPort  Port=6  Side=Right
  To : Outport
  wires:
  Bus Creator1/1 -> To/1  "m"
  Three-Phase V-I Measurement/1 -> [Vabc_bus]
  Three-Phase V-I Measurement/2 -> [Iabc]
  Data Type Conversion1/1 -> Mechanical Delay/1, Switch/2
  Three-Phase V-I Measurement1/1 -> [Vabc_line]
  Three-Phase V-I Measurement1/2 -> Terminator/1
  [Status] -> Bus Creator1/1  "Status"
  [Iabc] -> Bus Creator1/2  "Iabc"
  [Vabc_bus] -> Bus Creator1/3  "Vabc_bus"
  [Vabc_line] -> Bus Creator1/4  "Vabc_line"
  From/1 -> Data Type Conversion1/1
  Switch/1 -> Three-Phase Breaker (custom)/1, [Status]
  Mechanical Delay/1 -> Switch/1
  Constant2/1 -> Switch/3
  connections:
  c/RConn1 -- Three-Phase V-I Measurement1/RConn3
  b/RConn1 -- Three-Phase V-I Measurement1/RConn2
  a/RConn1 -- Three-Phase V-I Measurement1/RConn1
  C/RConn1 -- Three-Phase V-I Measurement/LConn3
  B/RConn1 -- Three-Phase V-I Measurement/LConn2
  Three-Phase V-I Measurement/LConn1 -- A/RConn1
  Three-Phase V-I Measurement1/LConn3 -- Three-Phase Breaker (custom)/RConn3 -- Three-Phase Series RLC Branch1/LConn3
  Three-Phase V-I Measurement1/LConn2 -- Three-Phase Breaker (custom)/RConn2 -- Three-Phase Series RLC Branch1/LConn2
  Three-Phase V-I Measurement1/LConn1 -- Three-Phase Breaker (custom)/RConn1 -- Three-Phase Series RLC Branch1/LConn1
  Three-Phase V-I Measurement/RConn3 -- Three-Phase Breaker (custom)/LConn3 -- Three-Phase Series RLC Branch/LConn3
  Three-Phase V-I Measurement/RConn2 -- Three-Phase Breaker (custom)/LConn2 -- Three-Phase Series RLC Branch/LConn2
  Three-Phase V-I Measurement/RConn1 -- Three-Phase Breaker (custom)/LConn1 -- Three-Phase Series RLC Branch/LConn1
  Three-Phase Series RLC Branch/RConn2 -- Three-Phase Series RLC Branch/RConn3 -- Ground/LConn1 -- Three-Phase Series RLC Branch/RConn1
  Three-Phase Series RLC Branch1/RConn2 -- Three-Phase Series RLC Branch1/RConn3 -- Ground1/LConn1 -- Three-Phase Series RLC Branch1/RConn1

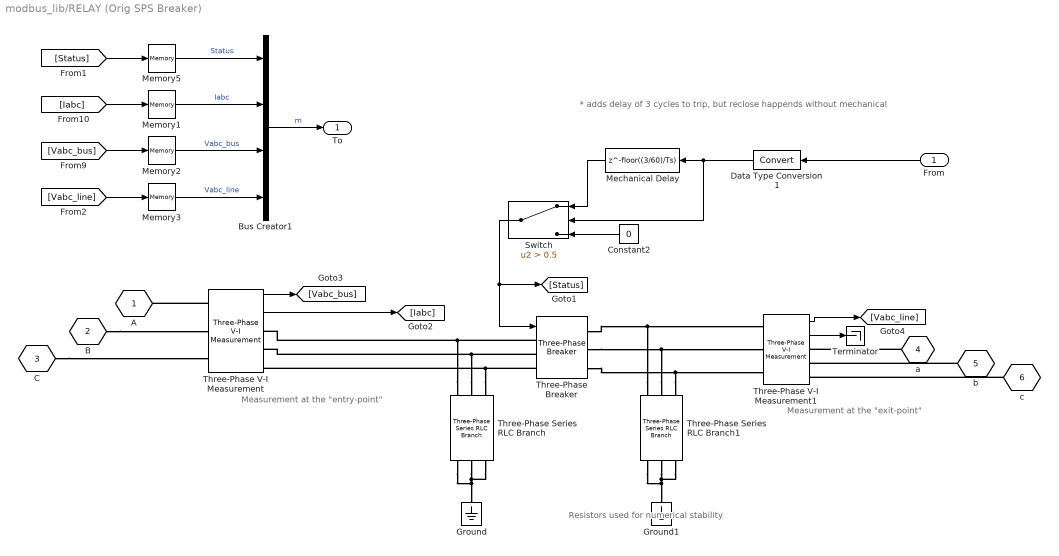
== system modbus_lib/RELAY (Orig SPS Breaker) ==
  note: * adds delay of 3 cycles to trip, but reclose happends without mechanical
  note: Measurement at the "exit-point"
  note: Measurement at the "entry-point"
  note: Resistors used for numerical stability
  From : Inport
  Bus Creator1 : BusCreator  Inputs=4
  Constant2 : Constant  Value=0
  Data Type Conversion1 : DataTypeConversion
  Ground : powerlib/Elements/Ground  LConnTagsString=a
  Ground1 : powerlib/Elements/Ground  LConnTagsString=a
  Mechanical Delay : Delay  DelayLength=floor((3/60)/Ts)  InitialCondition=1
  Memory{1..3,5} (4 alike) : Memory
  Switch : Switch  Criteria=u2 > Threshold  Threshold=0.5
  Terminator : Terminator
  Three-Phase Series RLC Branch : powerlib/Elements/Three-Phase Series RLC Branch  LConnTagsString=A|B|C  RConnTagsString=A|B|C  BranchType=R  Resistance=15E6  Inductance=1e-3  Capacitance=1e-6  Measurements=None
  Three-Phase Series RLC Branch1 : powerlib/Elements/Three-Phase Series RLC Branch  LConnTagsString=A|B|C  RConnTagsString=A|B|C  BranchType=R  Resistance=15E6  Inductance=1e-3  Capacitance=1e-6  Measurements=None
  Three-Phase V-I Measurement : powerlib/Measurements/Three-Phase V-I Measurement  VoltageMeasurement=phase-to-ground  SetLabelV=off  LabelV=Vabc  Vpu=off  VpuLL=off  CurrentMeasurement=yes  SetLabelI=off  LabelI=Iabc  Ipu=off  Pbase=100e6  Vbase=500e3  OutputType=Complex  PhasorSimulation=off  PSBequivalent=0
  Three-Phase V-I Measurement1 : powerlib/Measurements/Three-Phase V-I Measurement  VoltageMeasurement=phase-to-ground  SetLabelV=off  LabelV=Vabc  Vpu=off  VpuLL=off  CurrentMeasurement=yes  SetLabelI=off  LabelI=Iabc  Ipu=off  Pbase=100e6  Vbase=500e3  OutputType=Complex  PhasorSimulation=off  PSBequivalent=0
  Three-Phase Breaker : powerlib/Elements/Three-Phase Breaker  InitialState=closed  SwitchA=on  SwitchB=on  SwitchC=on  SwitchTimes="[1/60  5/60]"  External=on  BreakerResistance=1e-4  SnubberResistance=1E15  SnubberCapacitance=inf  Measurements=None
  A : PMIOPort  Tag=PMCPort  Port=1  Side=Left
  B : PMIOPort  Tag=PMCPort  Port=2  Side=Left
  C : PMIOPort  Tag=PMCPort  Port=3  Side=Left
  a : PMIOPort  Tag=PMCPort  Port=4  Side=Right
  b : PMIOPort  Tag=PMCPort  Port=5  Side=Right
  c : PMIOPort  Tag=PMCPort  Port=6  Side=Right
  To : Outport
  wires:
  Constant2/1 -> Switch/3
  Mechanical Delay/1 -> Switch/1
  Switch/1 -> [Status], Three-Phase Breaker/1
  From/1 -> Data Type Conversion1/1
  Memory3/1 -> Bus Creator1/4  "Vabc_line"
  Memory2/1 -> Bus Creator1/3  "Vabc_bus"
  Memory1/1 -> Bus Creator1/2  "Iabc"
  Memory5/1 -> Bus Creator1/1  "Status"
  Three-Phase V-I Measurement1/2 -> Terminator/1
  [Vabc_line] -> Memory3/1
  Three-Phase V-I Measurement1/1 -> [Vabc_line]
  [Vabc_bus] -> Memory2/1
  [Iabc] -> Memory1/1
  [Status] -> Memory5/1
  Data Type Conversion1/1 -> Switch/2, Mechanical Delay/1
  Three-Phase V-I Measurement/2 -> [Iabc]
  Three-Phase V-I Measurement/1 -> [Vabc_bus]
  Bus Creator1/1 -> To/1  "m"
  connections:
  Three-Phase Series RLC Branch1/RConn1 -- Ground1/LConn1 -- Three-Phase Series RLC Branch1/RConn3 -- Three-Phase Series RLC Branch1/RConn2
  Three-Phase Series RLC Branch/RConn1 -- Ground/LConn1 -- Three-Phase Series RLC Branch/RConn3 -- Three-Phase Series RLC Branch/RConn2
  Three-Phase Series RLC Branch/LConn1 -- Three-Phase V-I Measurement/RConn1 -- Three-Phase Breaker/LConn1
  Three-Phase Series RLC Branch/LConn2 -- Three-Phase V-I Measurement/RConn2 -- Three-Phase Breaker/LConn2
  Three-Phase Series RLC Branch/LConn3 -- Three-Phase V-I Measurement/RConn3 -- Three-Phase Breaker/LConn3
  Three-Phase Series RLC Branch1/LConn1 -- Three-Phase V-I Measurement1/LConn1 -- Three-Phase Breaker/RConn1
  Three-Phase Series RLC Branch1/LConn2 -- Three-Phase V-I Measurement1/LConn2 -- Three-Phase Breaker/RConn2
  Three-Phase Series RLC Branch1/LConn3 -- Three-Phase V-I Measurement1/LConn3 -- Three-Phase Breaker/RConn3
  Three-Phase V-I Measurement/LConn1 -- A/RConn1
  B/RConn1 -- Three-Phase V-I Measurement/LConn2
  C/RConn1 -- Three-Phase V-I Measurement/LConn3
  a/RConn1 -- Three-Phase V-I Measurement1/RConn1
  b/RConn1 -- Three-Phase V-I Measurement1/RConn2
  c/RConn1 -- Three-Phase V-I Measurement1/RConn3

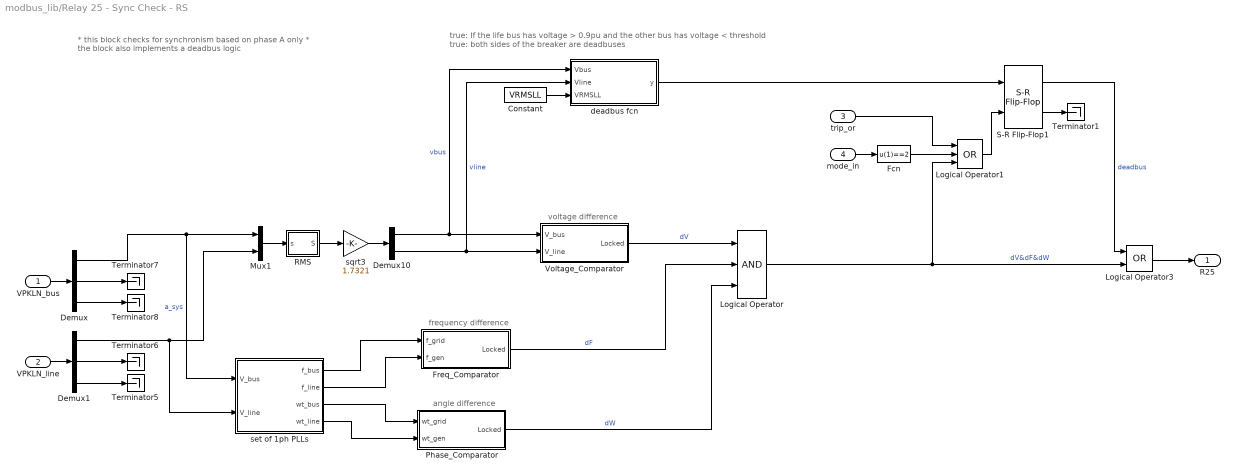
== system modbus_lib/Relay 25 - Sync Check - RS ==
  note: true: If the life bus has voltage > 0.9pu and the other bus has voltage < threshold
      | true: both sides of the breaker are deadbuses
  note: voltage difference
  note: frequency difference
  note: angle difference
  note: * this block checks for synchronism based on phase A only
      | * the block also implements a deadbus logic
  VPKLN_bus : Inport
  VPKLN_line : Inport  Port=2
  trip_or : Inport  Port=3
  mode_in : Inport  Port=4
  Constant : Constant  Value=VRMSLL
  Demux : Demux  Outputs=3
  Demux1 : Demux  Outputs=3
  Demux10 : Demux  Outputs=2
  Fcn : Fcn  Expr=u(1)==2
  Freq_Comparator : Subsystem
  Logical Operator : Logic  Inputs=3  AllPortsSameDT=off  OutDataTypeStr=boolean
  Logical Operator1 : Logic  Operator=OR  Inputs=3  AllPortsSameDT=off  OutDataTypeStr=boolean
  Logical Operator3 : Logic  Operator=OR  AllPortsSameDT=off  OutDataTypeStr=boolean
  Mux1 : Mux  Inputs=2
  Phase_Comparator : Subsystem
  RMS : Subsystem
  S-R Flip-Flop1 : simulink_extras/Flip Flops/S-R Flip-Flop  initial_condition=0
  Terminator{1,5..8} (5 alike) : Terminator
  Voltage_Comparator : Subsystem
  deadbus fcn : MATLAB Function  TreatAsAtomicUnit=on
  set of 1ph PLLs : Subsystem
  sqrt3 : Gain  Gain=1.7321
  R25 : Outport
  wires:
  Logical Operator/1 -> Logical Operator3/2, Logical Operator1/3  "dV&dF&dW"
  VPKLN_line/1 -> Demux1/1
  VPKLN_bus/1 -> Demux/1
  Demux/3 -> Terminator8/1
  Demux/2 -> Terminator7/1
  Demux1/3 -> Terminator5/1
  Demux1/2 -> Terminator6/1
  Demux1/1 -> set of 1ph PLLs/2(V_line), Mux1/2
  Demux/1 -> set of 1ph PLLs/1(V_bus), Mux1/1  "a_sys"
  Demux10/1 -> Voltage_Comparator/1(V_bus), deadbus fcn/1(Vbus)  "vbus"
  set of 1ph PLLs/1(f_bus) -> Freq_Comparator/1(f_grid)
  set of 1ph PLLs/2(f_line) -> Freq_Comparator/2(f_gen)
  set of 1ph PLLs/3(wt_bus) -> Phase_Comparator/1(wt_grid)
  set of 1ph PLLs/4(wt_line) -> Phase_Comparator/2(wt_gen)
  Demux10/2 -> Voltage_Comparator/2(V_line), deadbus fcn/2(Vline)  "vline"
  Voltage_Comparator/1(Locked) -> Logical Operator/1  "dV"
  Freq_Comparator/1(Locked) -> Logical Operator/2  "dF"
  Phase_Comparator/1(Locked) -> Logical Operator/3  "dW"
  RMS/1(S) -> sqrt3/1
  Mux1/1 -> RMS/1(s)
  sqrt3/1 -> Demux10/1
  Constant/1 -> deadbus fcn/3(VRMSLL)
  S-R Flip-Flop1/2 -> Terminator1/1
  Logical Operator3/1 -> R25/1
  S-R Flip-Flop1/1 -> Logical Operator3/1  "deadbus"
  deadbus fcn/1(y) -> S-R Flip-Flop1/1
  Logical Operator1/1 -> S-R Flip-Flop1/2
  trip_or/1 -> Logical Operator1/1
  mode_in/1 -> Fcn/1
  Fcn/1 -> Logical Operator1/2

== system modbus_lib/Relay w Comm ==
  Commands : Inport
  RELAY1 : modbus_lib/RELAY  Ts=Ts
  SEL_787_Relay : modbus_lib/SEL_787_Relay  bkrCtrl_enable=0  bkrCtrl_status=1  settings=[relay_sets(1, :)]  Ts=Ts
  A : PMIOPort  Port=1  Side=Left
  a : PMIOPort  Port=2  Side=Right
  B : PMIOPort  Port=3  Side=Left
  b : PMIOPort  Port=4  Side=Right
  C : PMIOPort  Port=5  Side=Left
  c : PMIOPort  Port=6  Side=Right
  RawMeasBus : Outport
  DerivedMeasBus : Outport  Port=2
  wires:
  RELAY1/1 -> SEL_787_Relay/1
  SEL_787_Relay/1 -> RawMeasBus/1, RELAY1/1
  Commands/1 -> SEL_787_Relay/2
  SEL_787_Relay/2 -> DerivedMeasBus/1
  connections:
  RELAY1/LConn1 -- A/RConn1
  RELAY1/RConn1 -- a/RConn1
  RELAY1/RConn3 -- c/RConn1
  RELAY1/LConn3 -- C/RConn1
  RELAY1/LConn2 -- B/RConn1
  RELAY1/RConn2 -- b/RConn1
